simulink model "pneumatics_controller"  (R2025a)
settings: Solver=VariableStepAuto  StartTime=0.0  StopTime=10.0  RelTol=1e-3
settings Model: Creator=adam  LastModifiedBy=adam

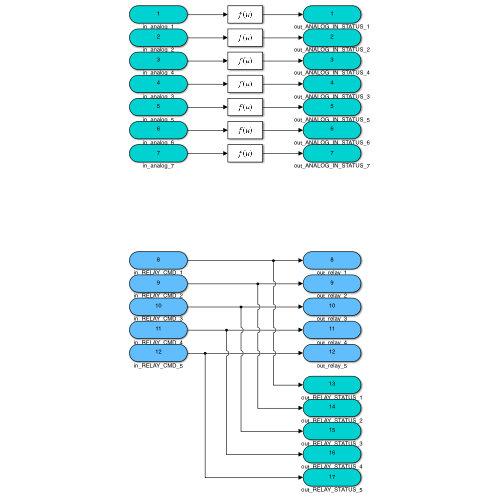
[thumbnail: Simulink's stored preview of the top-level diagram]
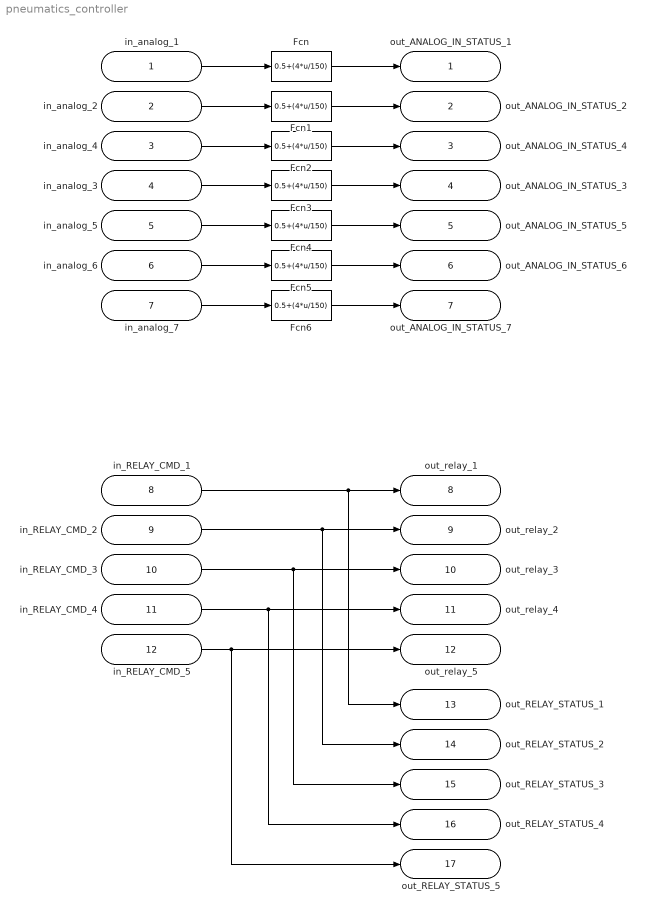
== system pneumatics_controller ==
  in_analog_1 : Inport
  in_analog_2 : Inport  Port=2
  in_analog_4 : Inport  Port=3
  in_analog_3 : Inport  Port=4
  in_analog_5 : Inport  Port=5
  in_analog_6 : Inport  Port=6
  in_analog_7 : Inport  Port=7
  in_RELAY_CMD_1 : Inport  Port=8
  in_RELAY_CMD_2 : Inport  Port=9
  in_RELAY_CMD_3 : Inport  Port=10
  in_RELAY_CMD_4 : Inport  Port=11
  in_RELAY_CMD_5 : Inport  Port=12
  Fcn{,1..6} (7 alike) : Fcn  Expr=0.5+(4*u/150)
  out_ANALOG_IN_STATUS_1 : Outport
  out_ANALOG_IN_STATUS_2 : Outport  Port=2
  out_ANALOG_IN_STATUS_4 : Outport  Port=3
  out_ANALOG_IN_STATUS_3 : Outport  Port=4
  out_ANALOG_IN_STATUS_5 : Outport  Port=5
  out_ANALOG_IN_STATUS_6 : Outport  Port=6
  out_ANALOG_IN_STATUS_7 : Outport  Port=7
  out_relay_1 : Outport  Port=8
  out_relay_2 : Outport  Port=9
  out_relay_3 : Outport  Port=10
  out_relay_4 : Outport  Port=11
  out_relay_5 : Outport  Port=12
  out_RELAY_STATUS_1 : Outport  Port=13
  out_RELAY_STATUS_2 : Outport  Port=14
  out_RELAY_STATUS_3 : Outport  Port=15
  out_RELAY_STATUS_4 : Outport  Port=16
  out_RELAY_STATUS_5 : Outport  Port=17
  wires:
  in_analog_1/1 -> Fcn/1
  in_analog_2/1 -> Fcn1/1
  in_analog_3/1 -> Fcn3/1
  in_analog_4/1 -> Fcn2/1
  in_analog_5/1 -> Fcn4/1
  in_analog_6/1 -> Fcn5/1
  in_analog_7/1 -> Fcn6/1
  in_RELAY_CMD_3/1 -> out_RELAY_STATUS_3/1, out_relay_3/1
  in_RELAY_CMD_1/1 -> out_RELAY_STATUS_1/1, out_relay_1/1
  in_RELAY_CMD_4/1 -> out_RELAY_STATUS_4/1, out_relay_4/1
  in_RELAY_CMD_5/1 -> out_RELAY_STATUS_5/1, out_relay_5/1
  in_RELAY_CMD_2/1 -> out_RELAY_STATUS_2/1, out_relay_2/1
  Fcn/1 -> out_ANALOG_IN_STATUS_1/1
  Fcn1/1 -> out_ANALOG_IN_STATUS_2/1
  Fcn2/1 -> out_ANALOG_IN_STATUS_4/1
  Fcn3/1 -> out_ANALOG_IN_STATUS_3/1
  Fcn5/1 -> out_ANALOG_IN_STATUS_6/1
  Fcn4/1 -> out_ANALOG_IN_STATUS_5/1
  Fcn6/1 -> out_ANALOG_IN_STATUS_7/1
